simulink model "LA1"  (R2019b)
settings: Solver=VariableStepAuto  StartTime=0.0  StopTime=10.0  RelTol=1e-3
undefined symbols (not defined in the file or in its folder): G, GG, kM, m, mG
libraries: Regler x3
settings Model: Creator=Admin  LastModifiedBy=Admin

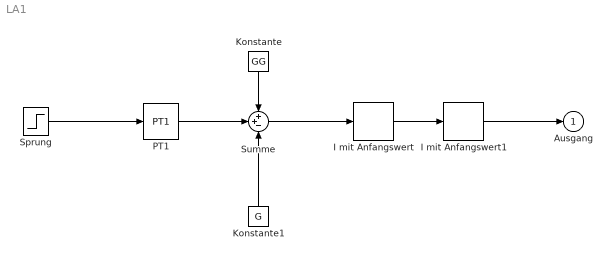
== system LA1 ==
  I mit Anfangswert : Regler/I mit Anfangswert  Ti=m+mG  u0=60
  I mit Anfangswert1 : Regler/I mit Anfangswert  Ti=1100  u0=60
  Konstante : Constant  Value=GG
  Konstante1 : Constant  Value=G
  PT1 : Regler/PT1  k=kM  T1=TM
  Sprung : Step  Time=0.000001  SampleTime=0
  Summe : Sum  Inputs=++-  SaturateOnIntegerOverflow=on  InputSameDT=on  OutDataTypeStr=Inherit: Same as first input
  Ausgang : Outport  VectorParamsAs1DForOutWhenUnconnected=off
  wires:
  Sprung/1 -> PT1/1
  I mit Anfangswert/1 -> I mit Anfangswert1/1
  I mit Anfangswert1/1 -> Ausgang/1
  Konstante/1 -> Summe/1
  PT1/1 -> Summe/2
  Konstante1/1 -> Summe/3
  Summe/1 -> I mit Anfangswert/1
